simulink model "Debounce_and_Healing"  (R2018a)
settings: Solver=FixedStepDiscrete  StartTime=0.0  StopTime=5  FixedStep=0.01  RelTol=1e-3
settings Model: SnapshotBufferSize=1000  Creator=Choaib ELMADI  LastModifiedBy=Choaib ELMADI

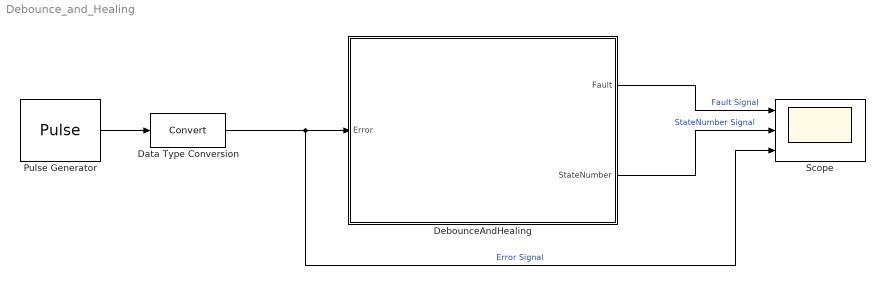
== system Debounce_and_Healing ==
  Data Type Conversion : DataTypeConversion
  DebounceAndHealing : Stateflow chart  TreatAsAtomicUnit=on
  Pulse Generator : DiscretePulseGenerator  PulseType=Time based  PulseWidth=90
  Scope : Scope  NumInputPorts=3
  wires:
  Pulse Generator/1 -> Data Type Conversion/1
  DebounceAndHealing/1(Fault) -> Scope/1  "Fault Signal"
  DebounceAndHealing/2(StateNumber) -> Scope/2  "StateNumber Signal"
  Data Type Conversion/1 -> DebounceAndHealing/1(Error), Scope/3  "Error Signal"

== stateflow chart Debounce_and_Healing/DebounceAndHealing ==
  state IDLE_STATE
    en:
    StateNumber = 1;
    Fault = false;
  state DEBOUNCE_STATE
    en:
    StateNumber = 2;
    Fault = false;
  state ACTIVE_STATE
    en:
    StateNumber = 3;
    Fault = true;
  (default) -> IDLE_STATE
  IDLE_STATE -> DEBOUNCE_STATE : [Error]
  DEBOUNCE_STATE -> IDLE_STATE [order 1] : [~Error]
  ACTIVE_STATE -> IDLE_STATE : after(20, tick)
  DEBOUNCE_STATE -> ACTIVE_STATE [order 2] : after(10, tick)
  data: Error input boolean; Fault output boolean; StateNumber output uint8
